simulink library "lib_decmp_Calib_tbm_supCtr_x8"  (R2020a)
settings: Solver=VariableStepAuto  StartTime=0.0  StopTime=10.0  RelTol=1e-3
settings Model: Creator=Administrator  LastModifiedBy=Administrator

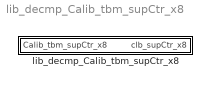
== system lib_decmp_Calib_tbm_supCtr_x8 ==
  lib_decmp_Calib_tbm_supCtr_x8 : Subsystem

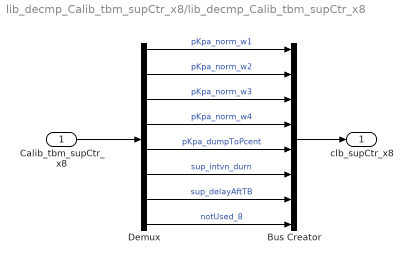
== system lib_decmp_Calib_tbm_supCtr_x8/lib_decmp_Calib_tbm_supCtr_x8 ==
  Calib_tbm_supCtr_x8 : Inport  OutDataTypeStr=single  PortDimensions=8
  Bus Creator : BusCreator  Inputs=8
  Demux : Demux  Outputs=8
  clb_supCtr_x8 : Outport  PortDimensions=8
  wires:
  Calib_tbm_supCtr_x8/1 -> Demux/1
  Demux/1 -> Bus Creator/1  "pKpa_norm_w1"
  Demux/2 -> Bus Creator/2  "pKpa_norm_w2"
  Demux/3 -> Bus Creator/3  "pKpa_norm_w3"
  Demux/4 -> Bus Creator/4  "pKpa_norm_w4"
  Bus Creator/1 -> clb_supCtr_x8/1
  Demux/5 -> Bus Creator/5  "pKpa_dumpToPcent"
  Demux/6 -> Bus Creator/6  "sup_intvn_durn"
  Demux/7 -> Bus Creator/7  "sup_delayAftTB"
  Demux/8 -> Bus Creator/8  "notUsed_8"
